simulink model "BBB_serial_basic"  (R2014b)
settings: Solver=ode3  StartTime=0.0  StopTime=10  RelTol=1e-3
settings Model: SimulationMode=external  Creator=Sebastian  LastModifiedBy=Sebastian
settings OptimizationCC: OptimizeModelRefInitCode=on  LifeSpan=1  MaxStackSize=64
settings HardwareCC: ProdLargestAtomicInteger=Long  ProdLargestAtomicFloat=Double  ProdEndianess=LittleEndian  ProdHWDeviceType=ARM Compatible->ARM Cortex
settings RTWCC: SystemTargetFile=ert.tlc  TLCOptions=-aInlineSetEventsForThisBaseRateFcn=TLC_FALSE -aSuppressMultiTaskScheduler=TLC_FALSE  TemplateMakefile=ert_default_tmf  Description=Embedded Coder  ProcessScript=ert_make_rtw_hook  Toolchain=Linaro Toolchain v4.8  BuildConfiguration=Specify
settings CodeAppCC: IgnoreCustomStorageClasses=off
settings ERTTargetCC: TargetLangStandard=C99 (ISO)  SupportNonInlinedSFcns=on  SupportVariableSizeSignals=on

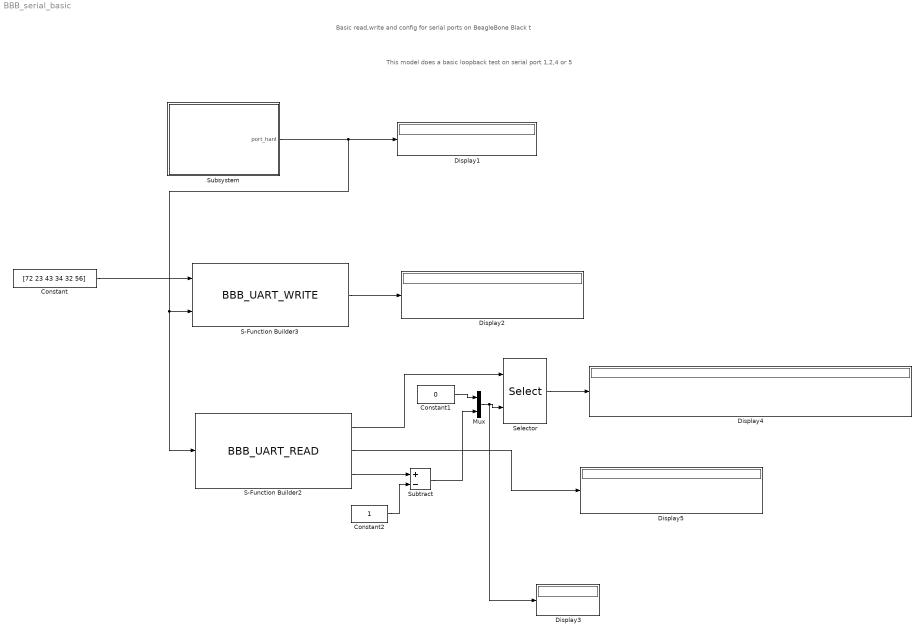
== system BBB_serial_basic ==
  note: This model does a basic loopback test on serial port 1,2,4 or 5
  note: Basic read,write and config for serial ports on BeagleBone Black t
  Constant : Constant  Value=[72 23 43 34 32 56]  OutDataTypeStr=uint8  SampleTime=1
  Constant1 : Constant  Value=0  OutDataTypeStr=int16
  Constant2 : Constant  OutDataTypeStr=int16
  Display{1..5} (5 alike) : Display
  Mux : Mux  Inputs=2
  S-Function Builder2 : S-Function  InitFcn=try, set_param(gcb,'FunctionName','BBB_UART_READ'), end  FunctionName=BBB_UART_READ  SFunctionModules=BBB_UART_READ_wrapper  EnableBusSupport=off  mask(S-Function Builder){}
      mask help: Simulink:masks:SFunctionBuilder_MD
      mask init:
      | val = [[.9  0.75 0.75 1 1 .9 .9 1]',[1 1 0.75 0.75 .9 .9 1 .9]'];try , sys = get_param(gcb,'SfunBuilderFcnName');if isempty(sys), sys = get_param(gcb,'FunctionName'); end,catch, sys = get_param(gcb,'FunctionName'); end
      settings: CopyFcn=set_param(gcbh,'LinkStatus','none')  PreSaveFcn=try, set_param(gcb,'FunctionName','BBB_UART_READ'), end  OpenFcn=sfunctionwizard(gcbh)
      mask Display: plot(val(:,1),val(:,2)),disp(sys), port_label('input',1,'port_handl'), port_label('output',1,'data'), port_label('output',2,'debug'), port_label('output',3,'bytes_read')
  S-Function Builder3 : S-Function  InitFcn=try, set_param(gcb,'FunctionName','BBB_UART_WRITE'), end  FunctionName=BBB_UART_WRITE  SFunctionModules=BBB_UART_WRITE_wrapper  EnableBusSupport=off  mask(S-Function Builder){}
      mask help: Simulink:masks:SFunctionBuilder_MD
      mask init: same as BBB_serial_basic/S-Function Builder2
      settings: CopyFcn=set_param(gcbh,'LinkStatus','none')  PreSaveFcn=try, set_param(gcb,'FunctionName','BBB_UART_WRITE'), end  OpenFcn=sfunctionwizard(gcbh)
      mask Display: plot(val(:,1),val(:,2)),disp(sys), port_label('input',1,'data'), port_label('input',2,'port_handl'), port_label('output',1,'debug')
  Selector : Selector  IndexMode=Zero-based  InputPortWidth=40  IndexOptions=Starting and ending indices (port)  Indices=[1 3]
  Subsystem : Subsystem  mask{portNbr=Uart 2}
      mask TypeOptions portNbr: Uart 1 | Uart 2 | Uart 4 | Uart 5
      mask Display:
      | gr_opt = get_param(gcb, 'portNbr');
      | fprintf('%s',gr_opt);
  Subtract : Sum  Inputs=+-
  wires:
  S-Function Builder2/2 -> Display5/1
  S-Function Builder3/1 -> Display2/1
  Constant/1 -> S-Function Builder3/1
  S-Function Builder2/1 -> Selector/1
  Selector/1 -> Display4/1
  Constant1/1 -> Mux/1
  Mux/1 -> Display3/1, Selector/2
  S-Function Builder2/3 -> Subtract/1
  Constant2/1 -> Subtract/2
  Subtract/1 -> Mux/2
  Subsystem/1(port_hanl) -> S-Function Builder2/1, S-Function Builder3/2, Display1/1

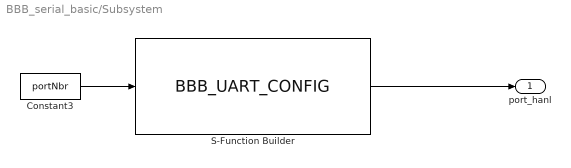
== system BBB_serial_basic/Subsystem ==
  Constant3 : Constant  Value=portNbr  OutDataTypeStr=int8
  S-Function Builder : S-Function  InitFcn=try, set_param(gcb,'FunctionName','BBB_UART_CONFIG'), end  FunctionName=BBB_UART_CONFIG  SFunctionModules=BBB_UART_CONFIG_wrapper  EnableBusSupport=off  mask(S-Function Builder){}
      mask help: Simulink:masks:SFunctionBuilder_MD
      mask init: same as BBB_serial_basic/S-Function Builder2
      settings: CopyFcn=set_param(gcbh,'LinkStatus','none')  PreSaveFcn=try, set_param(gcb,'FunctionName','BBB_UART_CONFIG'), end  OpenFcn=sfunctionwizard(gcbh)
      mask Display: plot(val(:,1),val(:,2)),disp(sys), port_label('input',1,'portNbr'), port_label('output',1,'port_handl')
  port_hanl : Outport
  wires:
  S-Function Builder/1 -> port_hanl/1
  Constant3/1 -> S-Function Builder/1
